simulink model "Windowlifts"  (R2017b)
settings: Solver=FixedStepDiscrete  StartTime=0.0  StopTime=inf  RelTol=1e-3
libraries: simulink x1
settings Model: Creator=macbook  LastModifiedBy=macbook

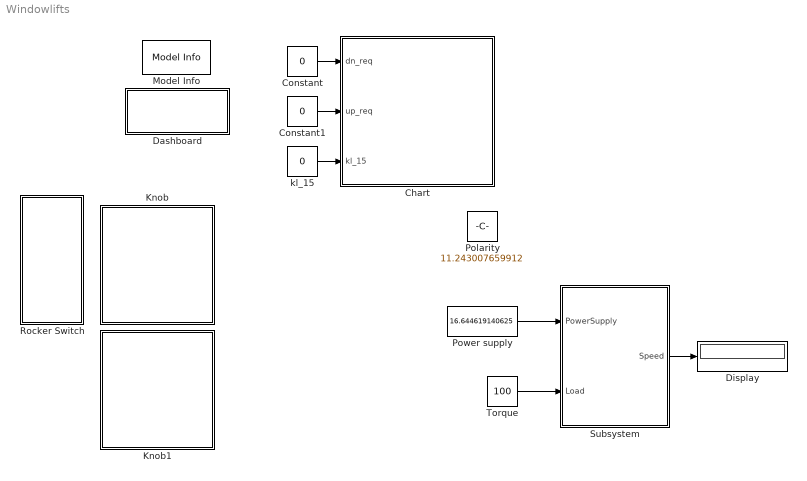
== system Windowlifts ==
  Chart : Stateflow chart  TreatAsAtomicUnit=on
  Constant : Constant  Value=0
  Constant1 : Constant  Value=0
  Dashboard : Subsystem  mask{Parameter2=<empty>}
      mask TypeOptions Parameter2: <empty>
  Display : Display
  Knob : Subsystem  DialogController=hmiCreateDDGDialog  IsWebBlock=on  mask(MWDashboardBlock){webBlockId=dafe5b38-9380-4eca-ae2b-aea756d26a10, webBlockType=continuousknob, ShowInLibBrowser=on, ShowInitialText=on, HMISrcModelName=example_1}
      mask prompts: webBlockId "WebBlock Id"; webBlockType "WebBlock Type"; HMISrcModelName "Source Model"
      mask help: SimulinkHMI:dialogs:ContinuousKnobDialogDesc
      mask Help: helpview([docroot '/mapfiles/simulink.map'], 'hmi_knob')
      mask Display:
      | if strcmp(get_param(bdroot(gcb),'BlockDiagramType'), 'library')
      |     image([(matlabroot) '/toolbox/simulink/hmi/icons/ContinuousKnob.png']);
      | end
  Knob1 : Subsystem  DialogController=hmiCreateDDGDialog  IsWebBlock=on  mask(MWDashboardBlock){webBlockId=805dc4ee-6b7c-4e6e-b950-217b83b8e70a, webBlockType=continuousknob, ShowInLibBrowser=on, ShowInitialText=on, HMISrcModelName=example_1}
      mask prompts: webBlockId "WebBlock Id"; webBlockType "WebBlock Type"; HMISrcModelName "Source Model"
      mask help: SimulinkHMI:dialogs:ContinuousKnobDialogDesc
      mask Help: helpview([docroot '/mapfiles/simulink.map'], 'hmi_knob')
      mask Display:
      | if strcmp(get_param(bdroot(gcb),'BlockDiagramType'), 'library')
      |     image([(matlabroot) '/toolbox/simulink/hmi/icons/ContinuousKnob.png']);
      | end
  Model Info : simulink/Model-Wide Utilities/Model Info  Frame=on  DisplayStringWithTags=Model Info  HorizontalTextAlignment=Center  LeftAlignmentValue=0.5
  Polarity : Constant  Value=11.243007659912
  Power supply : Constant  Value=16.644619140625
  Rocker Switch : Subsystem  DialogController=hmiCreateDDGDialog  IsWebBlock=on  mask(MWDashboardBlock){webBlockId=31a02f11-1852-4dac-a474-ed88ad0dbf04, webBlockType=rockerswitch, ShowInLibBrowser=on, ShowInitialText=on, HMISrcModelName=example_1}
      mask prompts: webBlockId "WebBlock Id"; webBlockType "WebBlock Type"; HMISrcModelName "Source Model"
      mask help: SimulinkHMI:dialogs:SwitchDialogDesc
      mask Help: helpview([docroot '/mapfiles/simulink.map'], 'hmi_rocker_switch')
      mask Display:
      | if strcmp(get_param(bdroot(gcb),'BlockDiagramType'), 'library')
      |     image([(matlabroot) '/toolbox/simulink/hmi/icons/RockerSwitch.png']);
      | end
  Subsystem : Subsystem
  Torque : Constant  Value=100
  kl_15 : Constant  Value=0
  wires:
  Constant/1 -> Chart/1(dn_req)
  Constant1/1 -> Chart/2(up_req)
  kl_15/1 -> Chart/3(kl_15)
  Subsystem/1(Speed) -> Display/1
  Power supply/1 -> Subsystem/1(PowerSupply)
  Torque/1 -> Subsystem/2(Load)

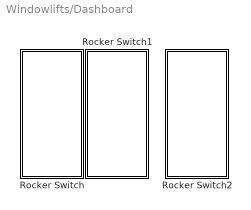
== system Windowlifts/Dashboard ==
  Rocker Switch : Subsystem  DialogController=hmiCreateDDGDialog  IsWebBlock=on  mask(MWDashboardBlock){webBlockId=025851f2-4a57-4a51-92c9-28208c54c957, webBlockType=rockerswitch, ShowInLibBrowser=on, ShowInitialText=on, HMISrcModelName=example_1}
      mask prompts: webBlockId "WebBlock Id"; webBlockType "WebBlock Type"; HMISrcModelName "Source Model"
      mask help: SimulinkHMI:dialogs:SwitchDialogDesc
      mask Help: helpview([docroot '/mapfiles/simulink.map'], 'hmi_rocker_switch')
      mask Display:
      | if strcmp(get_param(bdroot(gcb),'BlockDiagramType'), 'library')
      |     image([(matlabroot) '/toolbox/simulink/hmi/icons/RockerSwitch.png']);
      | end
  Rocker Switch1 : Subsystem  DialogController=hmiCreateDDGDialog  IsWebBlock=on  mask(MWDashboardBlock){webBlockId=e7ceb605-e41d-480e-a513-691243ba8675, webBlockType=rockerswitch, ShowInLibBrowser=on, ShowInitialText=on, HMISrcModelName=example_1}
      mask prompts: webBlockId "WebBlock Id"; webBlockType "WebBlock Type"; HMISrcModelName "Source Model"
      mask help: SimulinkHMI:dialogs:SwitchDialogDesc
      mask Help: helpview([docroot '/mapfiles/simulink.map'], 'hmi_rocker_switch')
      mask Display:
      | if strcmp(get_param(bdroot(gcb),'BlockDiagramType'), 'library')
      |     image([(matlabroot) '/toolbox/simulink/hmi/icons/RockerSwitch.png']);
      | end
  Rocker Switch2 : Subsystem  DialogController=hmiCreateDDGDialog  IsWebBlock=on  mask(MWDashboardBlock){webBlockId=4208986b-d946-4d67-8fd0-cf7385134c84, webBlockType=rockerswitch, ShowInLibBrowser=on, ShowInitialText=on, HMISrcModelName=example_1}
      mask prompts: webBlockId "WebBlock Id"; webBlockType "WebBlock Type"; HMISrcModelName "Source Model"
      mask help: SimulinkHMI:dialogs:SwitchDialogDesc
      mask Help: helpview([docroot '/mapfiles/simulink.map'], 'hmi_rocker_switch')
      mask Display:
      | if strcmp(get_param(bdroot(gcb),'BlockDiagramType'), 'library')
      |     image([(matlabroot) '/toolbox/simulink/hmi/icons/RockerSwitch.png']);
      | end

== system Windowlifts/Knob ==

== system Windowlifts/Knob1 ==

== system Windowlifts/Rocker Switch ==

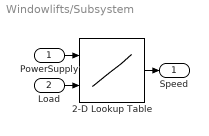
== system Windowlifts/Subsystem ==
  PowerSupply : Inport
  Load : Inport  Port=2
  2-D Lookup Table : Lookup_n-D  BreakpointsForDimension1=[0,6,10,12,14,16,20,24,32]  BreakpointsForDimension2=[0,15,45]  Table=reshape([0,500,1100,1500,1750,1850,1900,2000,2500,0,450,1000,1350,1500,1700,1800,1850,1850,0,300,900,1200,1300,1400,1550,1700,1700],9,3)  InternalRulePriority=Speed  OutDataTypeStr=int16  RndMeth=Simplest  InputSameDT=on
  Speed : Outport
  wires:
  2-D Lookup Table/1 -> Speed/1
  PowerSupply/1 -> 2-D Lookup Table/1
  Load/1 -> 2-D Lookup Table/2

== system Windowlifts/Dashboard/Rocker Switch ==

== system Windowlifts/Dashboard/Rocker Switch1 ==

== system Windowlifts/Dashboard/Rocker Switch2 ==

== stateflow chart Windowlifts/Chart ==
  note: Subsystem defines state of the system
  note: Subsystem defines the current output of the model
  note: Subsystem defines the kinematic of the drive
  state Logic [parallel]
    settings: executionOrder=1
    state up
      du:
      Current.ON;
      Kinematics.UP
    state bypass
      du:
      Current.OFF;
      Kinematics.IDLE
    state dn
      du:
      Current.ON;
      Kinematics.DN
    up -> bypass : [~up_req || dn_req || ~kl_15 ]
    bypass -> up [order 1] : [~dn_req && up_req]
    (default) -> bypass
    dn -> bypass : [~dn_req || up_req || ~kl_15]
    bypass -> dn [order 2] : [~up_req && dn_req]
  state Current [parallel]
    settings: executionOrder=2
    state current_on
    state current_off
    current_off -> current_on : ON
    current_on -> current_off : OFF
    (default) -> current_off
  state Kinematics [parallel]
    settings: executionOrder=3
    state idle
    state moving_down
    state moving_up
    (default) -> idle
    idle -> moving_down [order 1] : DN
    moving_down -> idle : IDLE
    idle -> moving_up [order 2] : UP
    moving_up -> idle : IDLE
  data: dn_req input; up_req input; kl_15 input
  events: ON local FUNCTION_CALL_EVENT; OFF local FUNCTION_CALL_EVENT; DN local FUNCTION_CALL_EVENT; UP local FUNCTION_CALL_EVENT; IDLE local FUNCTION_CALL_EVENT
